simulink model "test"  (R2020a)
settings: Solver=VariableStepAuto  StartTime=0.0  StopTime=t_sim  FixedStep=1  MaxStep=10  RelTol=1e-3
values from neighbouring files (symbols this model uses):
  max_thrust_acc = 0.01    [initial.m]
  mu = 3.986005*10^5    (= 398600.5)    [best_lambert.m]    (also in best_lambert_free.m; draft.m; dynamics.m = p.mu; initial.m)
libraries: simulink x1
settings Model: Creator=Mehdi  LastModifiedBy=Mehdi

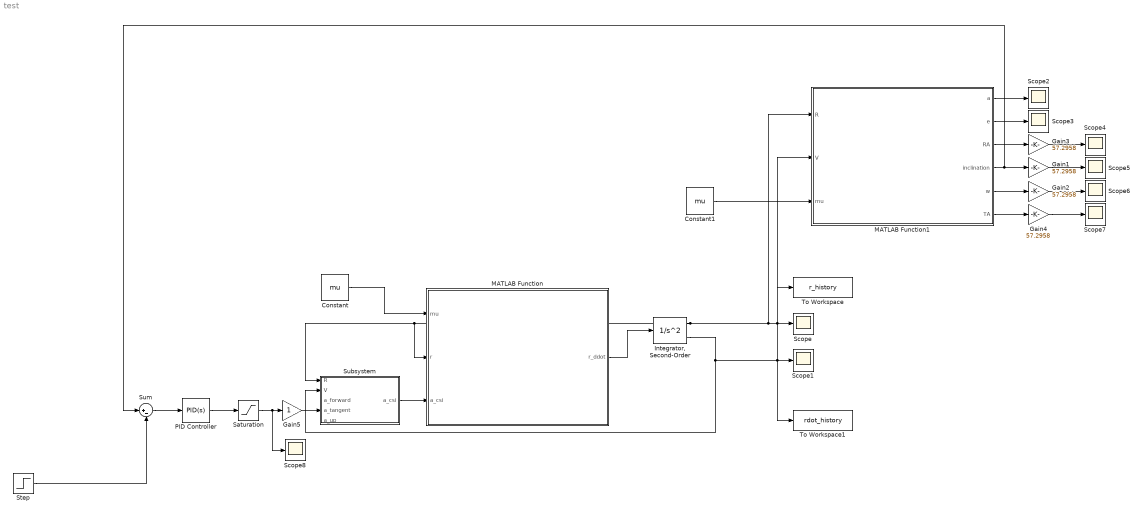
== system test ==
  Constant : Constant  Value=mu  VectorParams1D=off  SampleTime=-1
  Constant1 : Constant  Value=mu  VectorParams1D=off  SampleTime=-1
  Gain{1..4} (4 alike) : Gain  Gain=57.2958
  Gain5 : Gain
  "Integrator, Second-Order" : SecondOrderIntegrator  ICX=r0  ICDXDT=r_dot0
  MATLAB Function : MATLAB Function  TreatAsAtomicUnit=on
  MATLAB Function1 : MATLAB Function  TreatAsAtomicUnit=on
  PID Controller : simulink/Continuous/PID Controller  Controller=PID  Form=Parallel  TimeDomain=Continuous-time  UseExternalTs=off  SampleTime=-1  IntegratorMethod=Forward Euler  FilterMethod=Forward Euler  ControllerParametersSource=internal  P=0.001  I=0  D=0  UseFilter=on  N=100  TunerSelectOption=Frequency Response Based  InitialConditionSource=internal  InitialConditionForIntegrator=0  InitialConditionForFilter=0  DifferentiatorICPrevScaledInput=0  ExternalReset=none  TrackingMode=off  Kt=1  LimitOutput=off  UpperSaturationLimit=inf  LowerSaturationLimit=-inf  LinearizeAsGain=on  AntiWindupMode=none  Kb=1  POutMin=[]  POutMax=[]  IOutMin=[]  IOutMax=[]  DOutMin=[]  DOutMax=[]  NOutMin=[]  NOutMax=[]  SumOutMin=[]  SumOutMax=[]  SaturationOutMin=[]  SaturationOutMax=[]  PParamMin=[]  PParamMax=[]  IParamMin=[]  IParamMax=[]  DParamMin=[]  DParamMax=[]  NParamMin=[]  NParamMax=[]  KbParamMin=[]  KbParamMax=[]  KtParamMin=[]  KtParamMax=[]  KbOutMin=[]  KbOutMax=[]  KtOutMin=[]  KtOutMax=[]  IntegratorOutMin=[]  IntegratorOutMax=[]  FilterOutMin=[]  FilterOutMax=[]  SumI1OutMin=[]  SumI1OutMax=[]  SumI2OutMin=[]  SumI2OutMax=[]  SumI3OutMin=[]  SumI3OutMax=[]  SumI4OutMin=[]  SumI4OutMax=[]  SumDOutMin=[]  SumDOutMax=[]  DifferentiatorOutMin=[]  DifferentiatorOutMax=[]  FilterDiffOutCoefMin=[]  FilterDiffOutCoefMax=[]  ReciprocalOutMin=[]  ReciprocalOutMax=[]  SumDenOutMin=[]  SumDenOutMax=[]  SumNumOutMin=[]  SumNumOutMax=[]  DivideOutMin=[]  DivideOutMax=[]  UdiffTsProdOutMin=[]  UdiffTsProdOutMax=[]  NTsProdOutMin=[]  NTsProdOutMax=[]  UintegralTsProdOutMin=[]  UintegralTsProdOutMax=[]  UngainTsProdOutMin=[]  UngainTsProdOutMax=[]  IntegratorContinuousStateAttributes=''  IntegratorStateMustResolveToSignalObject=off  IntegratorRTWStateStorageClass=Auto  FilterContinuousStateAttributes=''  FilterStateMustResolveToSignalObject=off  FilterRTWStateStorageClass=Auto  ParallelPVariant=InternalParameters  IdealPVariant=Disabled  IVariant=InternalParameters  DVariant=InternalParameters  IntegratorVariant=Continuous  SatVariant=Disabled  AWVariant=Passthrough  PCopyVariant=Disabled  TRVariant=Disabled  FdbkBlocksVariant=Forward  IdealPFdbkVariant=Disabled  SatFdbkVariant=Disabled  DerivativeFilterVariant=ContFilter  NVariant=InternalParameters  NCopyVariant=Disabled  FilterICVariant=InternalICsFilter  IntegratorICVariant=InternalICs  ExternalResetVariant=Disabled  TRSumVariant=Passthrough  SumFdbkVariant=Disabled  SumVariant=Sum_PID  TsampFilterVariant=InternalTs  TsampNgainVariant=Passthrough  TsampIntegralVariant=Passthrough
  Saturation : Saturate  UpperLimit=max_thrust_acc  LowerLimit=-max_thrust_acc
  Scope{,1..8} (9 alike) : Scope
  Step : Step  Time=500  After=deg2rad(20)  SampleTime=0
  Subsystem : Subsystem
  Sum : Sum  Inputs=|+-
  To Workspace : ToWorkspace  VariableName=r_history  SaveFormat=Timeseries  SampleTime=-1
  To Workspace1 : ToWorkspace  VariableName=rdot_history  SaveFormat=Timeseries  SampleTime=-1
  wires:
  Constant/1 -> MATLAB Function/1(mu)
  "Integrator, Second-Order"/1 -> Subsystem/1(R), MATLAB Function/2(r), MATLAB Function1/1(R), To Workspace/1, Scope/1
  "Integrator, Second-Order"/2 -> MATLAB Function1/2(V), To Workspace1/1, Scope1/1, Subsystem/2(V)
  MATLAB Function/1(r_ddot) -> "Integrator, Second-Order"/1
  Constant1/1 -> MATLAB Function1/3(mu)
  MATLAB Function1/1(a) -> Scope2/1
  MATLAB Function1/2(e) -> Scope3/1
  MATLAB Function1/3(RA) -> Gain3/1
  MATLAB Function1/5(w) -> Gain2/1
  MATLAB Function1/6(TA) -> Gain4/1
  Subsystem/1(a_csi) -> MATLAB Function/3(a_csi)
  Step/1 -> Sum/2
  PID Controller/1 -> Saturation/1
  Sum/1 -> PID Controller/1
  Saturation/1 -> Scope8/1, Gain5/1
  MATLAB Function1/4(inclination) -> Sum/1, Gain1/1
  Gain1/1 -> Scope5/1
  Gain2/1 -> Scope6/1
  Gain4/1 -> Scope7/1
  Gain3/1 -> Scope4/1
  Gain5/1 -> Subsystem/4(a_tangent)

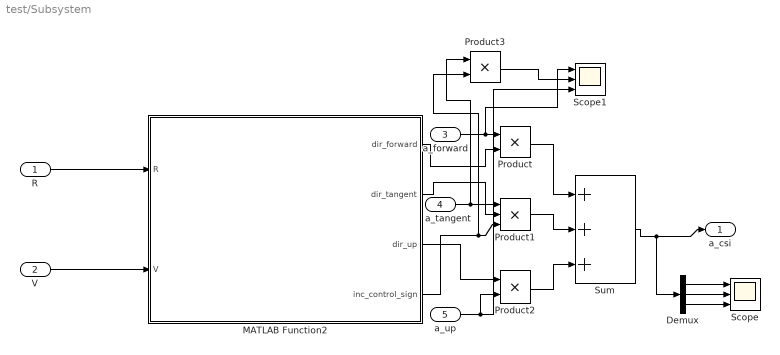
== system test/Subsystem ==
  R : Inport
  V : Inport  Port=2
  a_forward : Inport  Port=3
  a_tangent : Inport  Port=4
  a_up : Inport  Port=5
  Demux : Demux  Outputs=3
  MATLAB Function2 : MATLAB Function  TreatAsAtomicUnit=on
  Product : Product
  Product1 : Product  Inputs=3
  Product2 : Product
  Product3 : Product
  Scope : Scope  NumInputPorts=3
  Scope1 : Scope  NumInputPorts=3
  Sum : Sum  Inputs=+++
  a_csi : Outport
  wires:
  MATLAB Function2/1(dir_forward) -> Product/2
  Product/1 -> Sum/1
  Product1/1 -> Sum/2
  Product2/1 -> Sum/3
  R/1 -> MATLAB Function2/1(R)
  MATLAB Function2/2(dir_tangent) -> Product1/2
  V/1 -> MATLAB Function2/2(V)
  Sum/1 -> Demux/1, a_csi/1
  a_forward/1 -> Scope1/1, Product/1
  a_tangent/1 -> Product3/1, Product1/1
  a_up/1 -> Scope1/3, Product2/2
  MATLAB Function2/3(dir_up) -> Product2/1
  MATLAB Function2/4(inc_control_sign) -> Product3/2, Product1/3
  Demux/1 -> Scope/1
  Demux/2 -> Scope/2
  Demux/3 -> Scope/3
  Product3/1 -> Scope1/2

== matlab function test/MATLAB Function1 ==
  data: R input; V input; a output; mu input; e output; RA output; inclination output; w output; TA output
function [a, e, RA, inclination, w, TA] = oe_from_sv(R,V,mu)
%%%   This function computes the orbital elements (oe) from the 
%   state vector (R,V).
%   Based on Algorithm 4.2 from Orbital mechanics for engineering students,
%   2010, by H.D. Curtis 
%
%   INPUTS: 
%       R  = position vector state (km)
%       V  = velocity vector (km/s)
%       mu = gravitational parameter (km^3/s^2)
%   OUTPUT: 
%       oe = vector of orbital elements 
%
%   VARIABLES DESCRIPTION:
%       r, v - the magnitudes of R and V
%       vr   - radial velocity component (km/s)
%       H    - the angular momentum vector (km^2/s)
%       h    - the magnitude of H (km^2/s)
%       incl - inclination of the orbit (rad)
%       N    - the node line vector (km^2/s)
%       n    - the magnitude of N
%       cp   - cross product of N and R
%       RA   - right ascension of the ascending node (rad)
%       E    - eccentricity vector
%       e    - eccentricity (magnitude of E)
%       w    - argument of perigee (rad)
%       TA   - true anomaly (rad)
%       a    - semimajor axis (km)

%%% Calculate distance and speed
r = norm(R);
v = norm(V);

%% Calculate the radial velocity
vr = dot(R,V)/r;

%% Calculate the specific angular momentum 
H = cross(R,V);
h = norm(H);

%% Calculate the inclination 
inclination = acos(H(3)/h);

%% Calculate the node line N
N = cross([0 0 1],H);
n = norm(N);

eps = 1.e-10;
%% Calculate the right ascension the ascending node
if n ~= 0
    RA = acos(N(1)/n);
    if N(2) < 0
        RA = 2*pi - RA;
    end
else
    RA = 0;
end

%% Calculate the eccentricity vector and magnitude 
E = 1/mu*((v^2 - mu/r)*R - r*vr*V);
e = norm(E);

%% Calculate the argument of perigee 
if n ~= 0
    if e > eps
        w = acos(dot(N,E)/n/e);
    if E(3) < 0
        w = 2*pi - w;
    end
    else
        w = 0;
    end
else
    w = 0;
end

%% Calculate the true anomaly
if e > eps
    TA = acos(dot(E,R)/e/r);
    if vr < 0
        TA = 2*pi - TA;
    end
else
    cp = cross(N,R);
    if cp(3) >= 0
        TA = acos(dot(N,R)/n/r);
    else
        TA = 2*pi - acos(dot(N,R)/n/r);
    end
end
a = h^2/mu/(1 - e^2);

%% Orbial elements vector
% oe = [h e RA inclination w TA a];
end

== matlab function test/MATLAB Function ==
  data: mu input; r input; r_ddot output; a_csi input
function r_ddot = fcn(mu,r,a_csi)


r_ddot=zeros(3,1);
c1=-mu/(norm(r))^3;

r_ddot(1)=c1*r(1)+a_csi(1);
r_ddot(2)=c1*r(2)+a_csi(2);
r_ddot(3)=c1*r(3)+a_csi(3);

end

== matlab function test/Subsystem/MATLAB Function2 ==
  data: R input; V input; dir_forward output; dir_tangent output; dir_up output; inc_control_sign output
function [dir_forward,dir_tangent,dir_up,inc_control_sign] = spherical_dir(R,V)

dir_up=R/norm(R);
h=cross(R,V);
dir_tangent=h/norm(h);
dir_forward=cross(dir_tangent,dir_up);


r_perpendicular_to_surface=dot(dir_tangent,R);
inc_control_sign=-sign(r_perpendicular_to_surface);
% inc_control_sign=1;

end
